simulink model "quad_sim"  (R2017a)
settings: Solver=VariableStepAuto  StartTime=0.0  StopTime=10.0  RelTol=1e-3
libraries: simulink x1
settings Model: Creator=Bharath  LastModifiedBy=Bharath

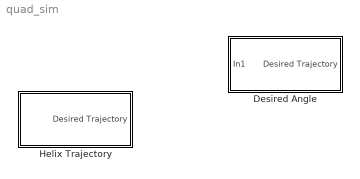
== system quad_sim ==
  Desired Angle : Subsystem
  Helix Trajectory : Subsystem

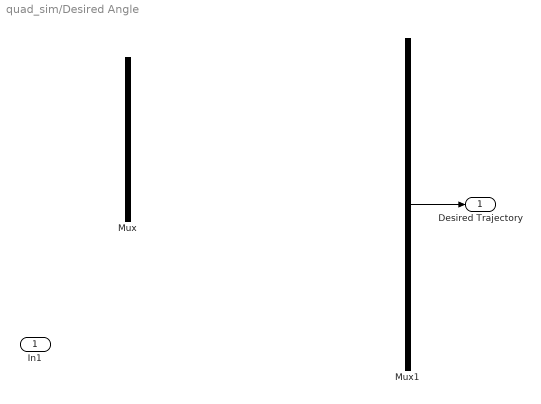
== system quad_sim/Desired Angle ==
  In1 : Inport
  Mux : Mux  Inputs=3
  Mux1 : Mux  Inputs=9
  Desired Trajectory : Outport
  wires:
  Mux1/1 -> Desired Trajectory/1

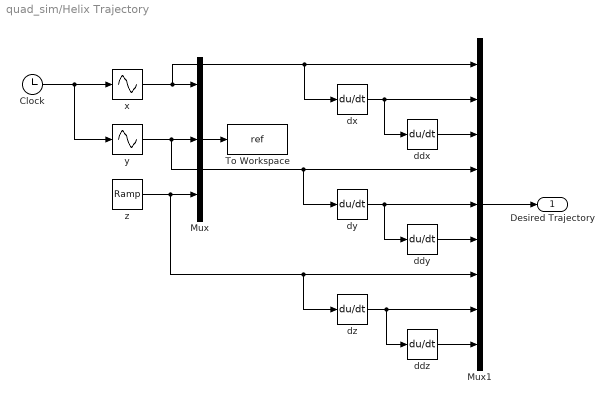
== system quad_sim/Helix Trajectory ==
  Clock : Clock
  Mux : Mux  Inputs=3
  Mux1 : Mux  Inputs=9
  To Workspace : ToWorkspace  VariableName=ref  SaveFormat=Timeseries  SampleTime=-1
  ddx : Derivative
  ddy : Derivative
  ddz : Derivative
  dx : Derivative
  dy : Derivative
  dz : Derivative
  x : Sin  TimeSource=Use external signal  Amplitude=8  Frequency=0.1  SampleTime=0
  y : Sin  TimeSource=Use external signal  Amplitude=8  Frequency=0.1  Phase=pi/2  SampleTime=0
  z : simulink/Sources/Ramp  slope=-0.2  start=0  X0=8
  Desired Trajectory : Outport
  wires:
  z/1 -> dz/1, Mux1/7, Mux/3
  dy/1 -> ddy/1, Mux1/5
  Mux/1 -> To Workspace/1
  dz/1 -> ddz/1, Mux1/8
  ddy/1 -> Mux1/6
  x/1 -> dx/1, Mux1/1, Mux/1
  y/1 -> dy/1, Mux1/4, Mux/2
  Mux1/1 -> Desired Trajectory/1
  dx/1 -> Mux1/2, ddx/1
  ddz/1 -> Mux1/9
  Clock/1 -> y/1, x/1
  ddx/1 -> Mux1/3
